simulink model "RightFront"  (R2020b)
settings: Solver=VariableStepAuto  StartTime=0.0  StopTime=10.0  RelTol=1e-3
undefined symbols (not defined in the file): sigbuilder_block
libraries: simulink x2
settings Model: Creator=Training  LastModifiedBy=Training

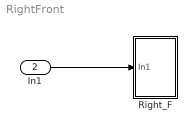
== system RightFront ==
  In1 : Inport  Port=2
  Right_F : Subsystem
  wires:
  In1/1 -> Right_F/1(In1)

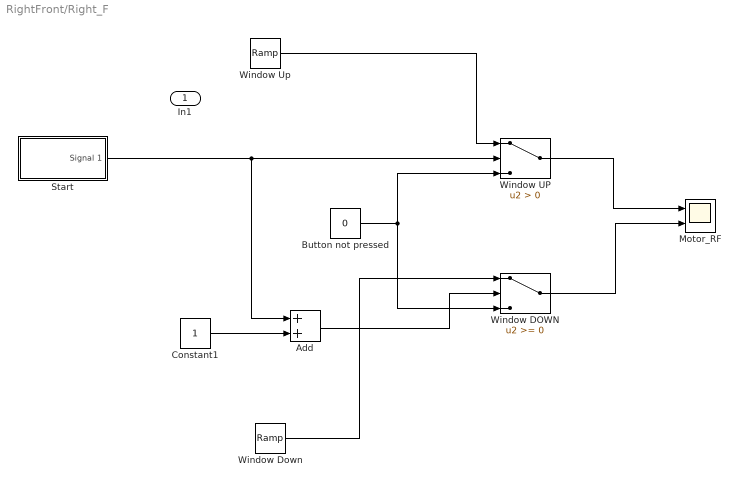
== system RightFront/Right_F ==
  In1 : Inport
  Add : Sum
  Button not pressed : Constant  Value=0
  Constant1 : Constant
  Motor_RF : Scope  NumInputPorts=2
  Start : Subsystem  Tag=STV Subsys  LoadFcn=sigbuilder_block('load');  StartFcn=sigbuilder_block('start');  StopFcn=sigbuilder_block('stop');  ClipboardFcn=sigbuilder_block('clipboard');  mask(Sigbuilder block){tuvar=[0:10]}
      mask help: Simulink:masks:SigbuilderBlock_MD
      mask init:
      | if ~strcmp(get_param(bdroot(gcbh),'SimulationStatus'),'stopped') tuvar = sigbuilder_block('maskInit'); end
      settings: CopyFcn=sigbuilder_block('copy');  DeleteFcn=sigbuilder_block('delete');  ModelCloseFcn=sigbuilder_block('modelClose');  PreSaveFcn=sigbuilder_block('preSave');  PauseFcn=sigbuilder_block('pause');  ContinueFcn=sigbuilder_block('continue');  NameChangeFcn=sigbuilder_block('namechange');  OpenFcn=sigbuilder_block('open',[437.6 199.2 550.4 400 ]);  CloseFcn=sigbuilder_block('close');
      mask Display: plot(0, 0, 100, 100,[2, 2, 32, 32, 2], [68, 8, 8, 68, 68],[32, 2], [38, 38], [32, 19, 2],[53, 60, 44], [32, 17, 17, 2],[16, 16, 31, 31]);txt = getActiveGroup(gcbh);text(2, 100, txt,'verticalAlignment', 'top');
  Window DOWN : Switch
  Window Down : simulink/Sources/Ramp  slope=1  start=0  InitialOutput=0
  Window UP : Switch  Criteria=u2 > Threshold
  Window Up : simulink/Sources/Ramp  slope=1  start=0  InitialOutput=0
  wires:
  Add/1 -> Window DOWN/2
  Button not pressed/1 -> Window UP/3, Window DOWN/3
  Constant1/1 -> Add/2
  Window Down/1 -> Window DOWN/1
  Window DOWN/1 -> Motor_RF/2
  Start/1(Signal 1) -> Add/1, Window UP/2
  Window Up/1 -> Window UP/1
  Window UP/1 -> Motor_RF/1

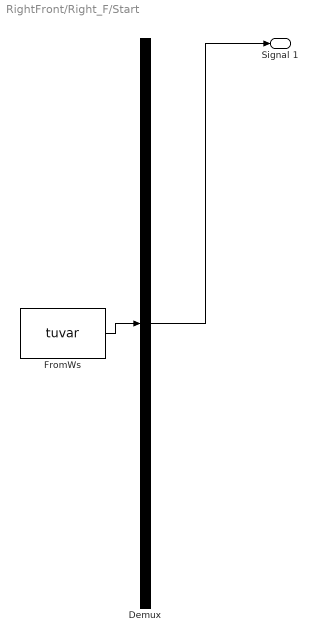
== system RightFront/Right_F/Start ==
  Demux : Demux  Tag=STV Demux  Outputs=1
      settings: DisplayOption=none
  FromWs : FromWorkspace  Tag=STV FromWs  VariableName=tuvar
      SigBuilderData=|
      | common.afterFinalStr = 'Extrapolate'
      | common.sampleTime = 0
      | dataSet.timeRange = [0 10]
      | dataSet.name = 'Group 1'
      | sbobj.Groups.Name = 'Group 1'
      | sbobj.Groups.Signals.Name = 'Signal 1'
      | sbobj.Groups.Signals.XData = [0 4 4 6 6 10]
      | sbobj.Groups.Signals.YData = [0 0 1 1 0 0]
  Signal 1 : Outport  Tag=STV Outport
  wires:
  Demux/1 -> Signal 1/1
  FromWs/1 -> Demux/1
